simulink model "Ex9_7model"  (R2013a)
settings: Solver=ode45  StartTime=0.0  StopTime=2  RelTol=1e-3
settings Model: Creator=John  LastModifiedBy=John
settings DataIOCC: SignalLoggingSaveFormat=ModelDataLogs
settings OptimizationCC: ExpressionDepthLimit=2147483647
settings DebuggingCC: FcnCallInpInsideContextMsg=UseLocalSettings  StrictBusMsg=Warning
settings GRTTargetCC: CombineOutputUpdateFcns=off  GRTInterface=on

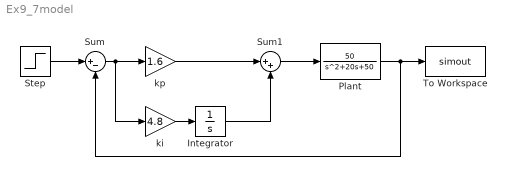
== system Ex9_7model ==
  Integrator : Integrator
  Plant : TransferFcn  Numerator=[50]  Denominator=[1 20 50]
  Step : Step  Time=0  SampleTime=0
  Sum : Sum  Inputs=|+-
  Sum1 : Sum  Inputs=|++
  To Workspace : ToWorkspace  VariableName=simout  SampleTime=-1
  ki : Gain  Gain=4.8
  kp : Gain  Gain=1.6
  wires:
  Plant/1 -> To Workspace/1, Sum/2
  Sum/1 -> kp/1, ki/1
  Step/1 -> Sum/1
  ki/1 -> Integrator/1
  Sum1/1 -> Plant/1
  Integrator/1 -> Sum1/2
  kp/1 -> Sum1/1
